simulink model "controlled_system"  (R2024b)
settings: Solver=VariableStepAuto  StartTime=0.0  StopTime=10.0  RelTol=1e-3
undefined symbols (not defined in the file): C, G, H_ext
settings Model: Creator=54238  LastModifiedBy=54238

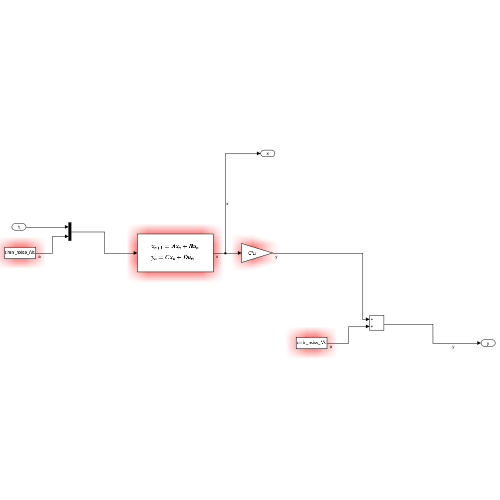
[thumbnail: Simulink's stored preview of the top-level diagram]
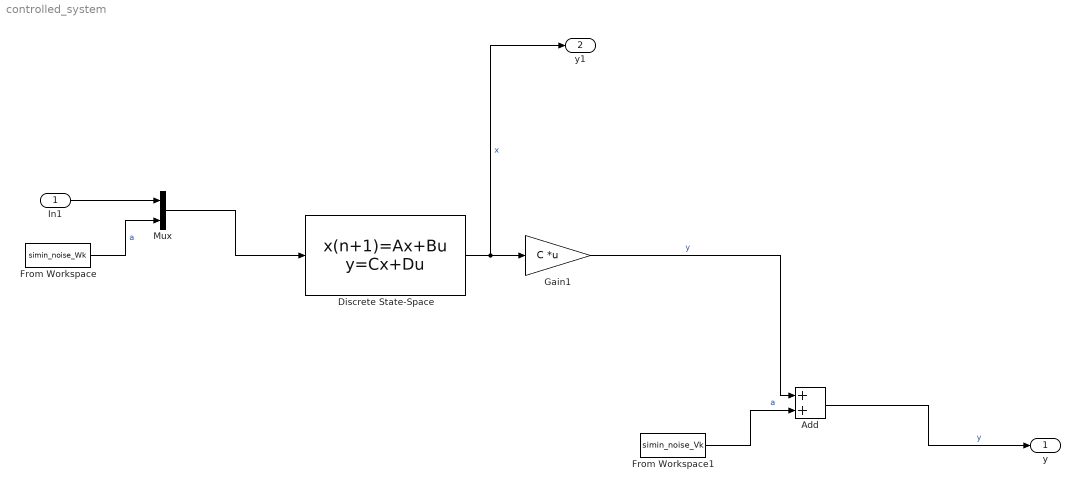
== system controlled_system ==
  In1 : Inport
  Add : Sum
  Discrete State-Space : DiscreteStateSpace  A=G  B=H_ext  C=[1 0 0 0;0 1 0 0;0 0 1 0;0 0 0 1]  D=[0 0 0 0 0 0 ;0 0 0 0 0 0 ;0 0 0 0 0 0 ;0 0 0 0 0 0 ]  InitialCondition=[0 0 0 0]  SampleTime=-1
  From Workspace : FromWorkspace  VariableName=simin_noise_Wk  SampleTime=-1
  From Workspace1 : FromWorkspace  VariableName=simin_noise_Vk  SampleTime=-1
  Gain1 : Gain  Gain=C  Multiplication=Matrix(K*u)
  Mux : Mux  Inputs=2
  y : Outport
  y1 : Outport  Port=2
  wires:
  Add/1 -> y/1  "y"
  Discrete State-Space/1 -> y1/1, Gain1/1  "x"
  From Workspace1/1 -> Add/2  "a"
  From Workspace/1 -> Mux/2  "a"
  Mux/1 -> Discrete State-Space/1
  Gain1/1 -> Add/1  "y"
  In1/1 -> Mux/1
